simulink subsystem "carModel"  (R2021b)
settings: Solver=VariableStepAuto  StartTime=0.0  StopTime=10.0  RelTol=1e-3
undefined symbols (not defined in the file or in its folder): sim_ic
settings Model: Creator=ze  LastModifiedBy=pedro

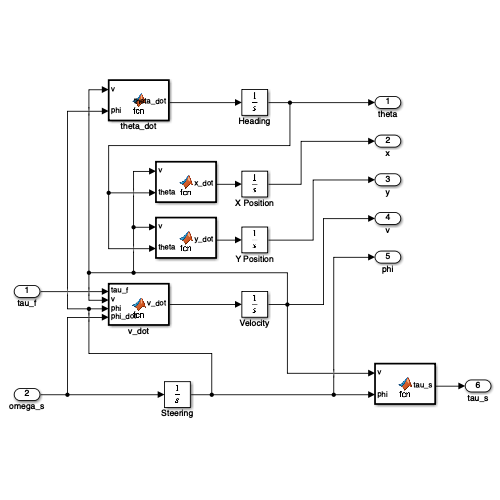
[thumbnail: Simulink's stored preview of the top-level diagram]
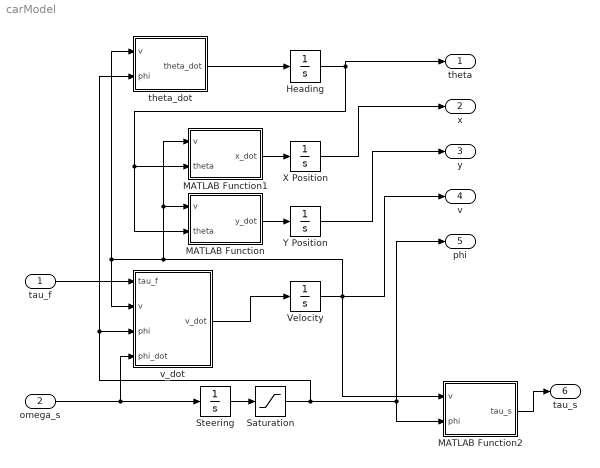
== system carModel ==
  tau_f : Inport
  omega_s : Inport  Port=2
  Heading : Integrator  InitialCondition=sim_ic.theta_0
  MATLAB Function : MATLAB Function  TreatAsAtomicUnit=on
  MATLAB Function1 : MATLAB Function  TreatAsAtomicUnit=on
  MATLAB Function2 : MATLAB Function  TreatAsAtomicUnit=on
  Saturation : Saturate  UpperLimit=pi/2 - 0.1  LowerLimit=-pi/2 + 0.1
  Steering : Integrator  InitialCondition=sim_ic.phi_0
  Velocity : Integrator  InitialCondition=sim_ic.v_0
  X Position : Integrator  InitialCondition=sim_ic.x_0
  Y Position : Integrator  InitialCondition=sim_ic.y_0
  theta_dot : MATLAB Function  TreatAsAtomicUnit=on
  v_dot : MATLAB Function  TreatAsAtomicUnit=on
  theta : Outport
  x : Outport  Port=2
  y : Outport  Port=3
  v : Outport  Port=4
  phi : Outport  Port=5
  tau_s : Outport  Port=6
  wires:
  omega_s/1 -> v_dot/4(phi_dot), Steering/1
  tau_f/1 -> v_dot/1(tau_f)
  Velocity/1 -> MATLAB Function2/1(v), MATLAB Function1/1(v), MATLAB Function/1(v), v_dot/2(v), theta_dot/1(v), v/1
  v_dot/1(v_dot) -> Velocity/1
  Steering/1 -> Saturation/1
  theta_dot/1(theta_dot) -> Heading/1
  MATLAB Function1/1(x_dot) -> X Position/1
  MATLAB Function/1(y_dot) -> Y Position/1
  Heading/1 -> MATLAB Function1/2(theta), MATLAB Function/2(theta), theta/1
  X Position/1 -> x/1
  Y Position/1 -> y/1
  MATLAB Function2/1(tau_s) -> tau_s/1
  Saturation/1 -> MATLAB Function2/2(phi), phi/1, v_dot/3(phi), theta_dot/2(phi)

== matlab function carModel/theta_dot ==
  data: v input; theta_dot output; phi input; car parameter
function theta_dot = fcn(v, phi, car)
    theta_dot = v*tan(phi)/car.L;

== matlab function carModel/v_dot ==
  data: tau_f input; v_dot output; v input; phi input; phi_dot input; car parameter
function v_dot = fcn(tau_f, v, phi, phi_dot, car)
    v_dot = 1/(car.M*car.r*cos(phi).^2) *(tau_f + car.M*car.r*v*sin(2*phi)*phi_dot);

== matlab function carModel/MATLAB Function ==
  data: v input; y_dot output; theta input
function y_dot = fcn(v, theta)
    y_dot = v*sin(theta);

== matlab function carModel/MATLAB Function1 ==
  data: v input; x_dot output; theta input
function x_dot = fcn(v, theta)
    x_dot = v*cos(theta);

== matlab function carModel/MATLAB Function2 ==
  data: v input; tau_s output; phi input; car parameter
function tau_s = fcn(v, phi, car)
    tau_s = -1/2 * (car.M*v.^2*sin(phi).^2);
